simulink model "LPV_Simula_SFUN"  (R2018a)
settings: Solver=VariableStepAuto  StartTime=0.0  StopTime=Tsim  RelTol=1e-3
values from neighbouring files (symbols this model uses):
  A = [1 0;a1';a2']    [test_sfun.m]
  A_ident = Modelo.A    [test_sfun.m]
  B = [0 0;b1';b2']    [test_sfun.m]
  B_ident = Modelo.B    [test_sfun.m]
  Ts = 0.1    [dados.mat]    (also in test_sfun.m)
  Tsim = 200    [test_sfun.m]
settings Model: Creator=root  LastModifiedBy=marcus

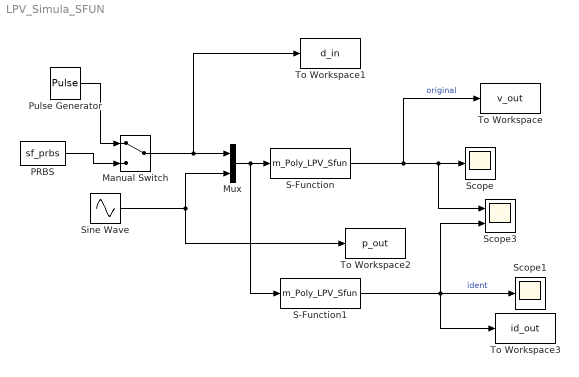
== system LPV_Simula_SFUN ==
  Manual Switch : ManualSwitch
  Mux : Mux  Inputs=2
  PRBS : S-Function  FunctionName=sf_prbs  Parameters=K,N,Ts  SFunctionDeploymentMode=off  EnableBusSupport=off  mask{K=0.3, N=7, Ts=0.12}
      mask prompts: K "Ganho (K):"; N "Número de Células (usar 5, 7 ou 10):"; Ts "Tempo de amostragem (seg):"
      mask Display: disp('P R B S')
  Pulse Generator : DiscretePulseGenerator  PulseType=Time based  Period=20  PulseWidth=50
  S-Function : S-Function  FunctionName=m_Poly_LPV_Sfun  Parameters=Ts,A,B  SFunctionDeploymentMode=off  EnableBusSupport=off
  S-Function1 : S-Function  FunctionName=m_Poly_LPV_Sfun  Parameters=Ts,A_ident,B_ident  SFunctionDeploymentMode=off  EnableBusSupport=off
  Scope : Scope
  Scope1 : Scope
  Scope3 : Scope  NumInputPorts=2
  Sine Wave : Sin  Amplitude=0.1  Bias=0.2  Frequency=2*pi/Tsim  SampleTime=0
  To Workspace : ToWorkspace  VariableName=v_out  SaveFormat=Timeseries  SampleTime=Ts
  To Workspace1 : ToWorkspace  VariableName=d_in  SaveFormat=Timeseries  SampleTime=Ts
  To Workspace2 : ToWorkspace  VariableName=p_out  SaveFormat=Timeseries  SampleTime=Ts
  To Workspace3 : ToWorkspace  VariableName=id_out  SaveFormat=Timeseries  SampleTime=Ts
  wires:
  Mux/1 -> S-Function1/1, S-Function/1
  Sine Wave/1 -> To Workspace2/1, Mux/2
  S-Function/1 -> Scope3/1, Scope/1, To Workspace/1  "original"
  Manual Switch/1 -> To Workspace1/1, Mux/1
  PRBS/1 -> Manual Switch/2
  Pulse Generator/1 -> Manual Switch/1
  S-Function1/1 -> To Workspace3/1, Scope3/2, Scope1/1  "ident"
